simulink library "EntertainmentLevelDetector"  (R2022b)
settings: Solver=VariableStepAuto  StartTime=0.0  StopTime=10.0  RelTol=1e-3
InitFcn:
  | EntertainmentLevelDetector_init;
values from neighbouring files (symbols this model uses):
  LD = struct('fastDecay', fastDecay, 'slowDecay', slowDecay,  	'holdTime', holdTime, 'holdMargin', holdMargin,      'min', min, 'max', max, 'maxSPL', maxSPL)    [EntertainmentLevelDetector_init.m]
undefined symbols (not defined in the file or in its folder): sys_defs
libraries: EntertainmentLevelDetectorBtc x1
settings Model: Creator=jb10849  LastModifiedBy=kl13806
settings SolverCC: AlgebraicLoopSolver=TrustRegion
settings DebuggingCC: UnconnectedInputMsg=warning  UnconnectedOutputMsg=warning  UnconnectedLineMsg=warning  SFMachineParentedDataDiag=warning  ArithmeticOperatorsInVariantConditions=warning
settings ModelReferenceCC: EnableRefExpFcnMdlSchedulingChecks=on
settings SFSimCC: SimUseLocalCustomCode=off  CustomCodeUndefinedFunction=UseInterfaceOnly
settings RTWCC: RTWUseLocalCustomCode=off  DLArmComputeVersion=19.05
settings CodeAppCC: StateflowObjectComments=on

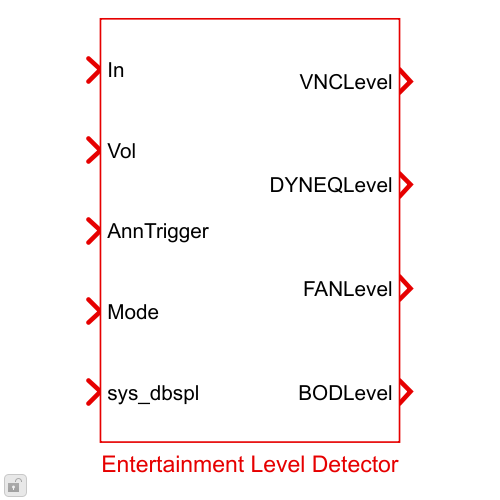
[thumbnail: Simulink's stored preview of the top-level diagram]
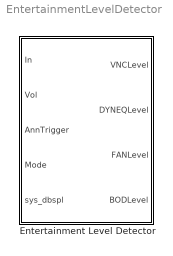
== system EntertainmentLevelDetector ==
  Entertainment Level Detector : Subsystem  mask(Level Detector for VNC, Dyanmic EQ, Fan and Boost-on-Demand){LD=LD, sys_defs=sys_defs}
      mask help: Level detector of entertainment audio in Audio Pilot.
      mask init:
      | InnerLinkConfig = EntertainmentLevelDetectorConfig;
      | InnerLinkConfig.FrameSize = sys_defs.frameSize;
      | InnerLinkConfig.Fs = sys_defs.Fs;
      | InnerLinkConfig.DefaultHoldMargin = LD.holdMargin;
      | InnerLinkConfig.DefaultMinVolDpSpl = LD.min;
      | InnerLinkConfig.DefaultMaxVolDbSpl = LD.max;
      | InnerLinkConfig.MaxSpl = LD.maxSPL;
      | 
      | % Use legacy api methods to back-compute original values
      | % (before decimation factor was introduced)
      | InnerLinkConfig.LegacyFastDecay(LD.fastDecay);
      | InnerLinkConfig.LegacySlowDecay(LD.slowDecay);
      | InnerLinkConfig.LegacyHoldTime(LD.holdTime);

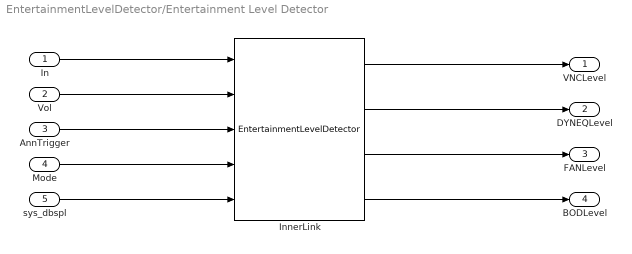
== system EntertainmentLevelDetector/Entertainment Level Detector ==
  In : Inport
  Vol : Inport  Port=2
  AnnTrigger : Inport  Port=3
  Mode : Inport  Port=4
  sys_dbspl : Inport  Port=5
  InnerLink : EntertainmentLevelDetectorBtc/EntertainmentLevelDetector  Config=InnerLinkConfig
  VNCLevel : Outport
  DYNEQLevel : Outport  Port=2
  FANLevel : Outport  Port=3
  BODLevel : Outport  Port=4
  wires:
  InnerLink/1 -> VNCLevel/1
  InnerLink/2 -> DYNEQLevel/1
  InnerLink/3 -> FANLevel/1
  InnerLink/4 -> BODLevel/1
  In/1 -> InnerLink/1
  Vol/1 -> InnerLink/2
  AnnTrigger/1 -> InnerLink/3
  Mode/1 -> InnerLink/4
  sys_dbspl/1 -> InnerLink/5
